simulink model "sim_Exp81_withFODPS"  (R2019b)
settings: Solver=VariableStepAuto  StartTime=0.0  StopTime=10.0  RelTol=1e-3
undefined symbols (not defined in the file): GP_den, GP_num
settings Model: Creator=sgxgong4  LastModifiedBy=xg
settings SFSimCC: CustomCodeUndefinedFunction=UseInterfaceOnly

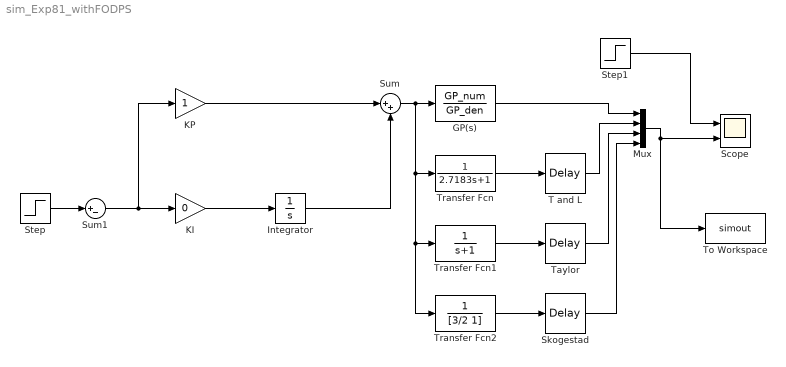
== system sim_Exp81_withFODPS ==
  GP(s) : TransferFcn  Numerator=GP_num  Denominator=GP_den
  Integrator : Integrator
  KI : Gain  Gain=0
  KP : Gain
  Mux : Mux
  Scope : Scope  NumInputPorts=2
  Skogestad : TransportDelay  DelayTime=1/2
  Step : Step  Time=0  SampleTime=0
  Step1 : Step  Time=0  SampleTime=0
  Sum : Sum  Inputs=|++
  Sum1 : Sum  Inputs=|+-
  "T and L " : TransportDelay  DelayTime=0.2817
  "Taylor " : TransportDelay
  To Workspace : ToWorkspace  VariableName=simout  SaveFormat=Structure With Time  SampleTime=-1
  Transfer Fcn : TransferFcn  Denominator=[2.7183 1]
  Transfer Fcn1 : TransferFcn  Denominator=[1 1]
  Transfer Fcn2 : TransferFcn  Denominator=[3/2 1]
  wires:
  KI/1 -> Integrator/1
  KP/1 -> Sum/1
  Integrator/1 -> Sum/2
  Sum1/1 -> KP/1, KI/1
  Step/1 -> Sum1/1
  Sum/1 -> Transfer Fcn2/1, Transfer Fcn1/1, Transfer Fcn/1, GP(s)/1
  GP(s)/1 -> Mux/1
  "T and L "/1 -> Mux/2
  Mux/1 -> To Workspace/1, Scope/2
  Transfer Fcn/1 -> "T and L "/1
  Transfer Fcn1/1 -> "Taylor "/1
  "Taylor "/1 -> Mux/3
  Transfer Fcn2/1 -> Skogestad/1
  Skogestad/1 -> Mux/4
  Step1/1 -> Scope/1
